simulink model "ncr18650b_thevenin"  (R2026a)
settings: Solver=ode45  StopTime=3600  RelTol=1e-4
settings Model: Creator=Razvan  LastModifiedBy=Razvan

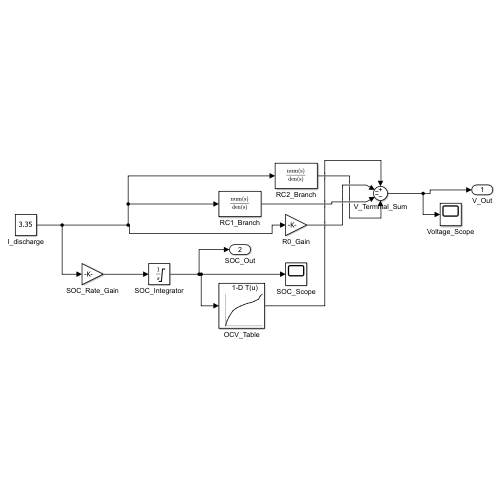
[thumbnail: Simulink's stored preview of the top-level diagram]
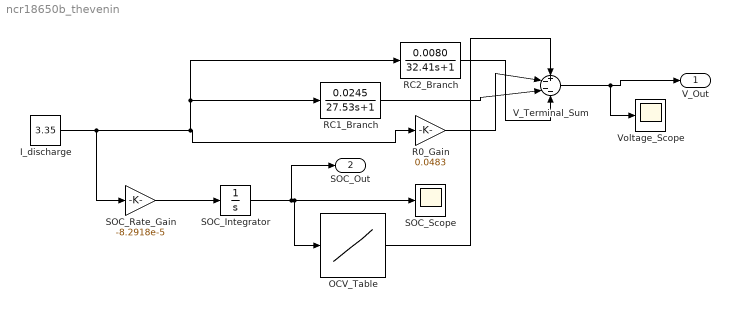
== system ncr18650b_thevenin ==
  I_discharge : Constant  Value=3.35
  OCV_Table : Lookup_n-D  NumberOfTableDimensions=1  BreakpointsForDimension1=[0 0.05 0.1 0.2 0.3 0.4 0.5 0.6 0.7 0.8 0.9 0.95 1.0]  Table=[2.65 2.90 3.10 3.40 3.55 3.65 3.72 3.78 3.83 3.90 4.00 4.12 4.25]  InternalRulePriority=Speed  RndMeth=Simplest
  R0_Gain : Gain  Gain=0.0483
  RC1_Branch : TransferFcn  Numerator=[0.0245]  Denominator=[27.53 1]
  RC2_Branch : TransferFcn  Numerator=[0.0080]  Denominator=[32.41 1]
  SOC_Integrator : Integrator  InitialCondition=1  LimitOutput=on  UpperSaturationLimit=1  LowerSaturationLimit=0
  SOC_Rate_Gain : Gain  Gain=-8.2918e-5
  SOC_Scope : Scope
  V_Terminal_Sum : Sum  Inputs=+---
  Voltage_Scope : Scope
  V_Out : Outport  VectorParamsAs1DForOutWhenUnconnected=off
  SOC_Out : Outport  Port=2  VectorParamsAs1DForOutWhenUnconnected=off
  wires:
  I_discharge/1 -> RC2_Branch/1, RC1_Branch/1, R0_Gain/1, SOC_Rate_Gain/1
  SOC_Rate_Gain/1 -> SOC_Integrator/1
  SOC_Integrator/1 -> SOC_Scope/1, OCV_Table/1, SOC_Out/1
  OCV_Table/1 -> V_Terminal_Sum/1
  R0_Gain/1 -> V_Terminal_Sum/2
  RC1_Branch/1 -> V_Terminal_Sum/3
  RC2_Branch/1 -> V_Terminal_Sum/4
  V_Terminal_Sum/1 -> V_Out/1, Voltage_Scope/1
